simulink model "Combination_Test"  (R2020b)
settings: Solver=VariableStepAuto  StartTime=0.0  StopTime=10.0  RelTol=1e-3
libraries: PB_Library_Master x2, Lib_Solve_SSNRSolverJC_TMATS x2
settings Model: Creator=gfretti  LastModifiedBy=nbutler2
settings SFSimCC: CustomCodeUndefinedFunction=UseInterfaceOnly

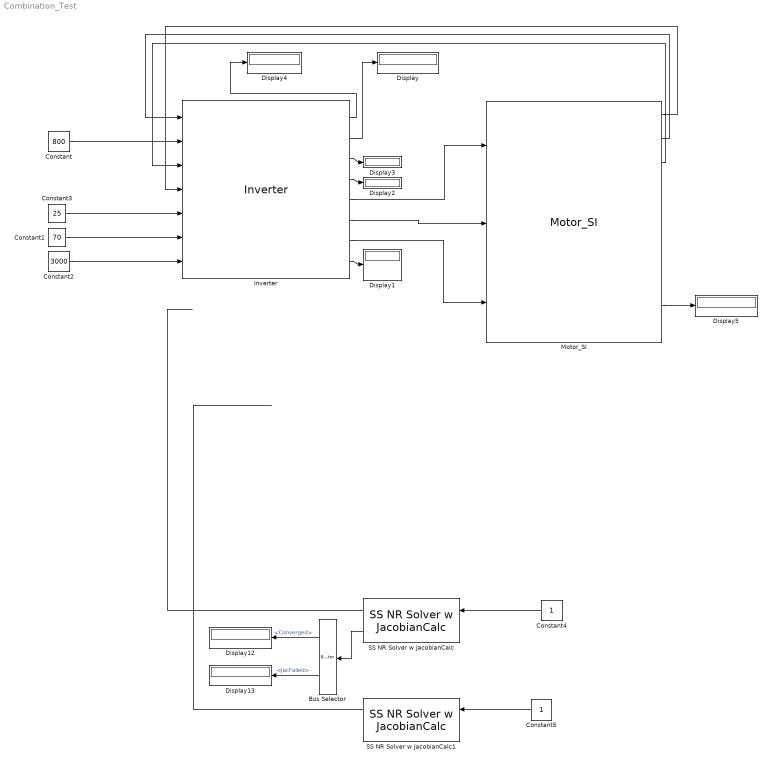
== system Combination_Test ==
  Bus Selector : BusSelector  OutputSignals=Converged,JacFailed
  Constant : Constant  Value=800
  Constant1 : Constant  Value=70
  Constant2 : Constant  Value=3000
  Constant3 : Constant  Value=25
  Constant4 : Constant
  Constant5 : Constant
  Display{,1..5,12..13} (8 alike) : Display
  Inverter : PB_Library_Master/Inverter  T_M=[25 175]  u_D_M=[1.16666666666667 0.999999999999998]  u_ce0_M=[0.971428571428571 0.848275862068965]  R_c_M=[0.0285714285714286 0.0551724137931034]  R_D_M=[0.0238095238095238 0.0294117647058824]  E0_M=[6.00000000000002e-05 6.00000000000002e-05]  E1_M=[5.6e-05 5.6e-05]  f_sw_M=20000  L_s_M=0.00115  P_max_I=22000  V_phase_I=400  f_sw_I=0  L_s_I=.00086+0.00029
  Motor_SI : PB_Library_Master/Motor_SI  pp=2  flux_m=0.57773  R_s=0.032  L_s=0.00115  P_Fe_Nom=904.3614  S_nom=3000  T_nom=70  P_out_max=22000  I_max=36.5  P_in_max=30000  T_max=80  MassEst_M=136.5892  Poles_i=4  R_s_i=.032  L_s_i=.00086+0.00029  S_nom_i=3000  T_nom_i=70  P_out_max_i=22000  I_max_i=36.5  P_in_max_i=30000  K_i=121  V_nom_i=368  T_max_i=80  CalculatePFe=Compute iron losses automatically  P_Fe_Nom_i=0  I_nom_i=36.5  PF_nom_i=0.99  P_Fe_Calc_Flag=1
  SS NR Solver w JacobianCalc : Lib_Solve_SSNRSolverJC_TMATS/SS NR Solver w JacobianCalc  SJac_Per_M=[-0.01;0.01]  SNR_IC_M=10  SNR_DX_M=100  SNR_Mx_M=100000  SNR_Mn_M=0.00001  SJacobianAttempts_M=20000  Cond_Limits_M=0.01
  SS NR Solver w JacobianCalc1 : Lib_Solve_SSNRSolverJC_TMATS/SS NR Solver w JacobianCalc  SJac_Per_M=[-0.01;0.01]  SNR_IC_M=150  SNR_DX_M=100  SNR_Mx_M=100000  SNR_Mn_M=0.00001  SJacobianAttempts_M=20000  Cond_Limits_M=0.01
  wires:
  Inverter/5 -> Motor_SI/1
  Inverter/6 -> Motor_SI/2
  Inverter/7 -> Motor_SI/3
  Motor_SI/2 -> Inverter/1
  Constant1/1 -> Inverter/6
  Constant2/1 -> Inverter/7
  Motor_SI/1 -> Inverter/4
  Motor_SI/3 -> Inverter/3
  Constant/1 -> Inverter/2
  Inverter/2 -> Display/1
  Inverter/8 -> Display1/1
  Inverter/4 -> Display2/1
  Inverter/3 -> Display3/1
  Inverter/1 -> Display4/1
  Motor_SI/9 -> Display5/1
  Constant3/1 -> Inverter/5
  ? -> SS NR Solver w JacobianCalc/2
  SS NR Solver w JacobianCalc1/1 -> ?
  SS NR Solver w JacobianCalc/1 -> ?
  Bus Selector/1 -> Display12/1  "<Converged>"
  Bus Selector/2 -> Display13/1  "<JacFailed>"
  SS NR Solver w JacobianCalc/2 -> Bus Selector/1
  Constant5/1 -> SS NR Solver w JacobianCalc1/1
  ? -> SS NR Solver w JacobianCalc1/2
  Constant4/1 -> SS NR Solver w JacobianCalc/1
